simulink model "nlmodel_3D_11"  (R2022a)
settings: Solver=ode45  StartTime=0.0  StopTime=10  RelTol=1e-3  EnableMultiTasking=on
undefined symbols (not defined in the file or in its folder): Ad, Bd, eps0, eps0dot, K, Kr, lam0, lam0dot, p1, p10, p2, p3, p4, p5, p6, p7, p8, p9, R_10, ro0, ro0dot, u0, x0
settings Model: Creator=giusgiordano  LastModifiedBy=Ccm
settings SolverCC: AlgebraicLoopSolver=TrustRegion
settings DataIOCC: LimitDataPoints=on  SaveFormat=Array  SignalLoggingSaveFormat=ModelDataLogs  ReturnWorkspaceOutputs=off
settings OptimizationCC: ExpressionDepthLimit=2147483647  LifeSpan=inf
settings DebuggingCC: UnderspecifiedInitializationDetection=Classic  MergeDetectMultiDrivingBlocksExec=none  SolverPrmCheckMsg=warning  FcnCallInpInsideContextMsg=warning  UnconnectedInputMsg=warning  UnconnectedOutputMsg=warning  UnconnectedLineMsg=warning  StateNameClashWarn=warning  SFUnexpectedBacktrackingDiag=warning  SFNoUnconditionalDefaultTransitionDiag=warning  SFExecutionAtInitializationDiag=none  SFMachineParentedDataDiag=warning  ArithmeticOperatorsInVariantConditions=warning
settings HardwareCC: ProdBitPerPointer=32  ProdBitPerSizeT=32  ProdBitPerPtrDiffT=32  ProdLargestAtomicFloat=None  ProdIntDivRoundTo=Undefined  ProdEndianess=Unspecified  ProdWordSize=32  ProdHWDeviceType=32-bit Generic
settings ModelReferenceCC: PropagateSignalLabelsOutOfModel=off
settings SFSimCC: SimUseLocalCustomCode=off  CustomCodeUndefinedFunction=UseInterfaceOnly
settings RTWCC: RTWUseLocalCustomCode=off
settings CodeAppCC: StateflowObjectComments=on
settings GRTTargetCC: TargetLangStandard=C89/C90 (ANSI)  CombineOutputUpdateFcns=off  GRTInterface=on
settings ConfigComp: CovMetricSettings=dw  CovSaveCumulativeToWorkspaceVar=on  CovSaveSingleToWorkspaceVar=on  CovExternalEMLEnable=off

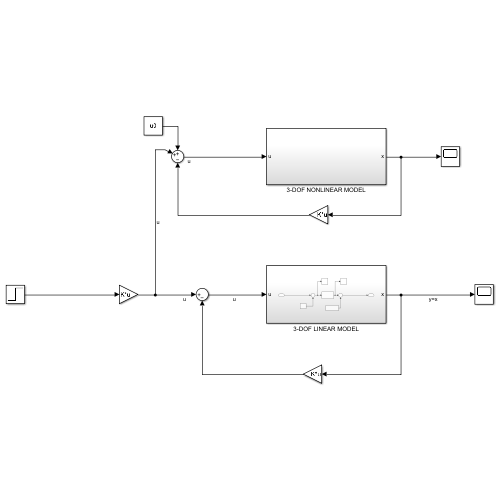
[thumbnail: Simulink's stored preview of the top-level diagram]
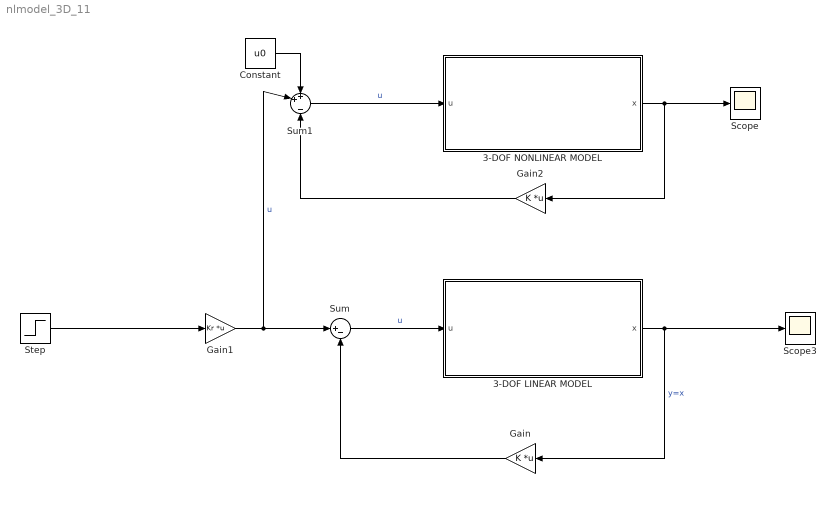
== system nlmodel_3D_11 ==
  3-DOF LINEAR MODEL : Subsystem
  3-DOF NONLINEAR MODEL : Subsystem
  Constant : Constant  Value=u0
  Gain : Gain  Gain=K  Multiplication=Matrix(K*u)
  Gain1 : Gain  Gain=Kr  Multiplication=Matrix(K*u)
  Gain2 : Gain  Gain=K  Multiplication=Matrix(K*u)
  Scope : Scope
  Scope3 : Scope
  Step : Step  Time=0  After=R_10  SampleTime=0
  Sum : Sum  Inputs=|+-
  Sum1 : Sum  Inputs=++|-
  wires:
  Sum/1 -> 3-DOF LINEAR MODEL/1(u)  "u"
  Gain1/1 -> Sum1/2, Sum/1  "u"
  Gain/1 -> Sum/2
  3-DOF LINEAR MODEL/1(x) -> Gain/1, Scope3/1  "y=x"
  Step/1 -> Gain1/1
  Constant/1 -> Sum1/1
  Sum1/1 -> 3-DOF NONLINEAR MODEL/1(u)  "u"
  Gain2/1 -> Sum1/3
  3-DOF NONLINEAR MODEL/1(x) -> Gain2/1, Scope/1

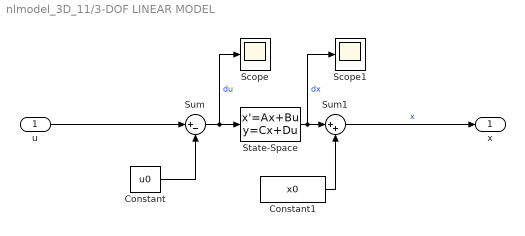
== system nlmodel_3D_11/3-DOF LINEAR MODEL ==
  u : Inport
  Constant : Constant  Value=u0
  Constant1 : Constant  Value=x0
  Scope : Scope
  Scope1 : Scope
  State-Space : StateSpace  A=Ad  B=Bd  C=eye(size(Ad))  D=zeros(size(Bd))  InitialCondition=x0  ContinuousStateAttributes={'eps','ro','lam','epsdot','rodot','lamdot'}
  Sum : Sum  Inputs=|+-
  Sum1 : Sum  Inputs=|++
  x : Outport
  wires:
  Constant1/1 -> Sum1/2
  Constant/1 -> Sum/2
  Sum/1 -> Scope/1, State-Space/1  "du"
  State-Space/1 -> Scope1/1, Sum1/1  "dx"
  u/1 -> Sum/1
  Sum1/1 -> x/1  "x"

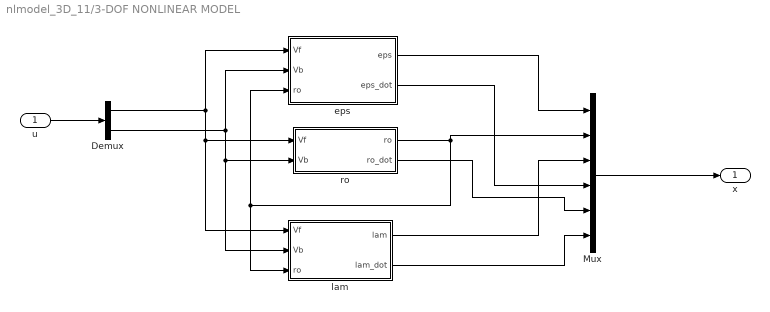
== system nlmodel_3D_11/3-DOF NONLINEAR MODEL ==
  u : Inport
  Demux : Demux  Outputs=2
  Mux : Mux  Inputs=6
  eps : Subsystem
  lam : Subsystem
  ro : Subsystem
  x : Outport
  wires:
  u/1 -> Demux/1
  Demux/1 -> eps/1(Vf), ro/1(Vf), lam/1(Vf)
  Demux/2 -> eps/2(Vb), ro/2(Vb), lam/2(Vb)
  ro/1(ro) -> Mux/2, eps/3(ro), lam/3(ro)
  Mux/1 -> x/1
  eps/1(eps) -> Mux/1
  lam/1(lam) -> Mux/3
  eps/2(eps_dot) -> Mux/4
  ro/2(ro_dot) -> Mux/5
  lam/2(lam_dot) -> Mux/6

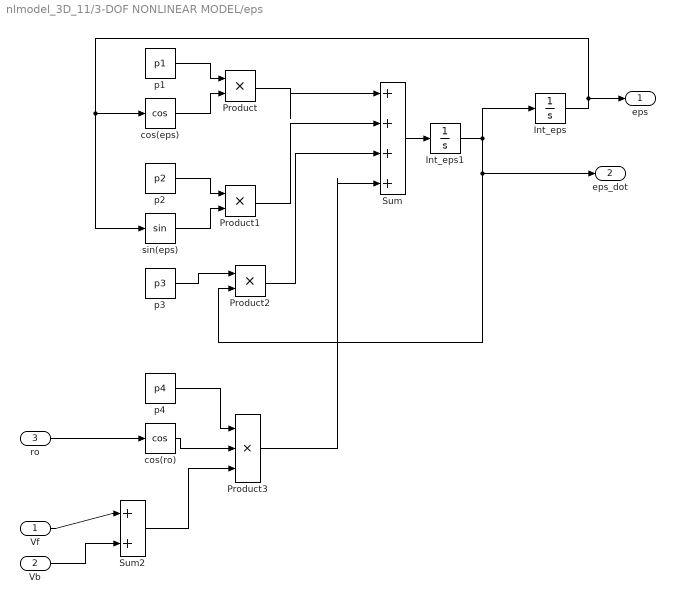
== system nlmodel_3D_11/3-DOF NONLINEAR MODEL/eps ==
  Vf : Inport
  Vb : Inport  Port=2
  ro : Inport  Port=3
  Int_eps : Integrator  InitialCondition=eps0  ContinuousStateAttributes='eps'
  Int_eps1 : Integrator  InitialCondition=eps0dot  ContinuousStateAttributes='epsdot'
  Product : Product  RndMeth=Zero
  Product1 : Product  RndMeth=Zero
  Product2 : Product  RndMeth=Zero
  Product3 : Product  Inputs=3  RndMeth=Zero
  Sum : Sum  Inputs=|++++
  Sum2 : Sum  Inputs=|++
  cos(eps) : Trigonometry  Operator=cos
  cos(ro) : Trigonometry  Operator=cos
  p1 : Constant  Value=p1
  p2 : Constant  Value=p2
  p3 : Constant  Value=p3
  p4 : Constant  Value=p4
  sin(eps) : Trigonometry
  eps : Outport
  eps_dot : Outport  Port=2
  wires:
  Int_eps/1 -> cos(eps)/1, sin(eps)/1, eps/1
  p1/1 -> Product/1
  cos(eps)/1 -> Product/2
  Product/1 -> Sum/1
  p2/1 -> Product1/1
  sin(eps)/1 -> Product1/2
  Product1/1 -> Sum/2
  p3/1 -> Product2/1
  Product2/1 -> Sum/3
  p4/1 -> Product3/1
  cos(ro)/1 -> Product3/2
  ro/1 -> cos(ro)/1
  Product3/1 -> Sum/4
  Sum/1 -> Int_eps1/1
  Int_eps1/1 -> Product2/2, eps_dot/1, Int_eps/1
  Vf/1 -> Sum2/1
  Vb/1 -> Sum2/2
  Sum2/1 -> Product3/3

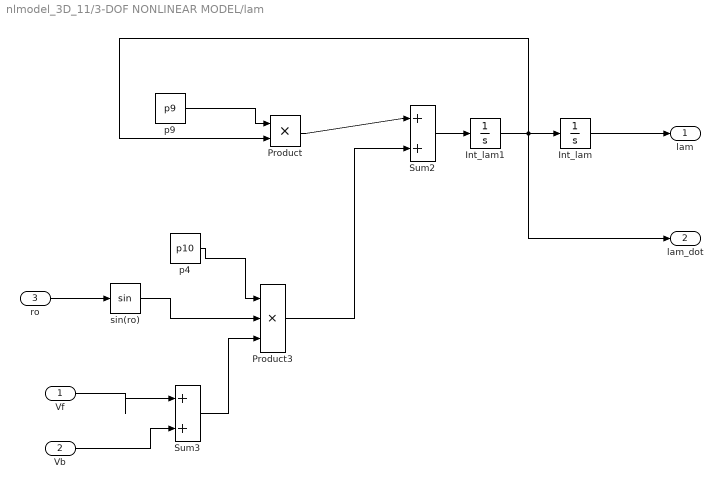
== system nlmodel_3D_11/3-DOF NONLINEAR MODEL/lam ==
  Vf : Inport
  Vb : Inport  Port=2
  ro : Inport  Port=3
  Int_lam : Integrator  InitialCondition=lam0  ContinuousStateAttributes='lam'
  Int_lam1 : Integrator  InitialCondition=lam0dot  ContinuousStateAttributes='lamdot'
  Product : Product  RndMeth=Zero
  Product3 : Product  Inputs=3  RndMeth=Zero
  Sum2 : Sum  Inputs=|++
  Sum3 : Sum  Inputs=|++
  p4 : Constant  Value=p10
  p9 : Constant  Value=p9
  sin(ro) : Trigonometry
  lam : Outport
  lam_dot : Outport  Port=2
  wires:
  Int_lam/1 -> lam/1
  p9/1 -> Product/1
  p4/1 -> Product3/1
  sin(ro)/1 -> Product3/2
  ro/1 -> sin(ro)/1
  Product/1 -> Sum2/1
  Sum2/1 -> Int_lam1/1
  Product3/1 -> Sum2/2
  Int_lam1/1 -> lam_dot/1, Product/2, Int_lam/1
  Vf/1 -> Sum3/1
  Vb/1 -> Sum3/2
  Sum3/1 -> Product3/3

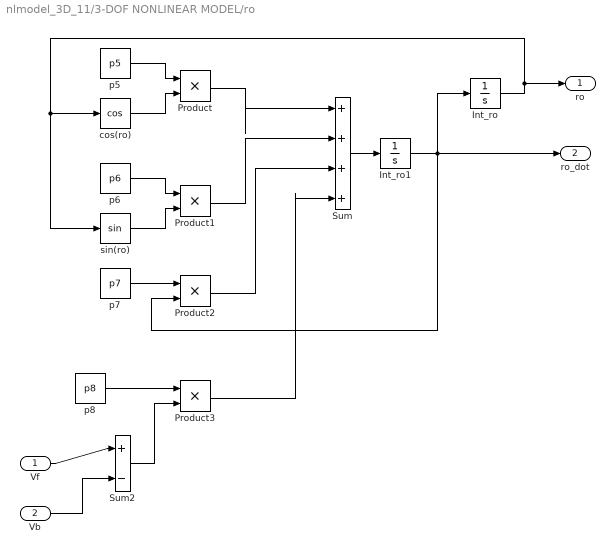
== system nlmodel_3D_11/3-DOF NONLINEAR MODEL/ro ==
  Vf : Inport
  Vb : Inport  Port=2
  Int_ro : Integrator  InitialCondition=ro0  ContinuousStateAttributes='ro'
  Int_ro1 : Integrator  InitialCondition=ro0dot  ContinuousStateAttributes='rodot'
  Product{,1..3} (4 alike) : Product  RndMeth=Zero
  Sum : Sum  Inputs=|++++
  Sum2 : Sum  Inputs=|+-
  cos(ro) : Trigonometry  Operator=cos
  p5 : Constant  Value=p5
  p6 : Constant  Value=p6
  p7 : Constant  Value=p7
  p8 : Constant  Value=p8
  sin(ro) : Trigonometry
  ro : Outport
  ro_dot : Outport  Port=2
  wires:
  Int_ro/1 -> cos(ro)/1, sin(ro)/1, ro/1
  p5/1 -> Product/1
  cos(ro)/1 -> Product/2
  Product/1 -> Sum/1
  p6/1 -> Product1/1
  sin(ro)/1 -> Product1/2
  Product1/1 -> Sum/2
  p7/1 -> Product2/1
  Product2/1 -> Sum/3
  p8/1 -> Product3/1
  Product3/1 -> Sum/4
  Int_ro1/1 -> Product2/2, ro_dot/1, Int_ro/1
  Sum/1 -> Int_ro1/1
  Vf/1 -> Sum2/1
  Vb/1 -> Sum2/2
  Sum2/1 -> Product3/2
